simulink model "Ganancia1Toworkspace"  (R2018a)
settings: Solver=ode4  StartTime=0.0  StopTime=10.0  FixedStep=0.05  RelTol=1e-3
settings Model: Creator=adtenla  LastModifiedBy=adtenla

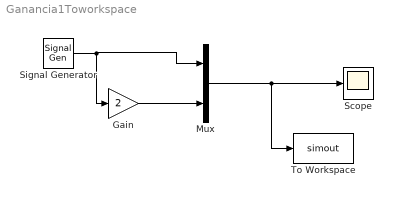
== system Ganancia1Toworkspace ==
  Gain : Gain  Gain=2
  Mux : Mux  Inputs=2
  Scope : Scope
  Signal Generator : SignalGenerator  Frequency=6  Units=rad/sec
  To Workspace : ToWorkspace  VariableName=simout  SampleTime=-1
  wires:
  Signal Generator/1 -> Mux/1, Gain/1
  Gain/1 -> Mux/2
  Mux/1 -> To Workspace/1, Scope/1
